simulink model "simulinkModel"  (R2021b)
settings: Solver=FixedStepAuto  StartTime=0.0  StopTime=50  FixedStep=0.05  RelTol=1e-3
model workspace (MAT data in the model file):
  R_wheel = 0.0565
  W = 0.055
  WD = 0.573125555665
  a = 0.306622172281
  b = 0.228377827719
  c = 0.38
  l = 0.535
  m = 13.4973333333
  m_LF = 2867.66666667
  m_LR = 3883.33333333
  m_RF = 2894
  m_RR = 3852.33333333
  m_f = 5761.66666667
  m_r = 7735.66666667
undefined symbols (not defined in the file or in its folder): sigbuilder_block
libraries: slpidlib x1
settings Model: PacingRate=0.100000  Creator=Mikeh  LastModifiedBy=20212181
settings DebuggingCC: SignalInfNanChecking=error

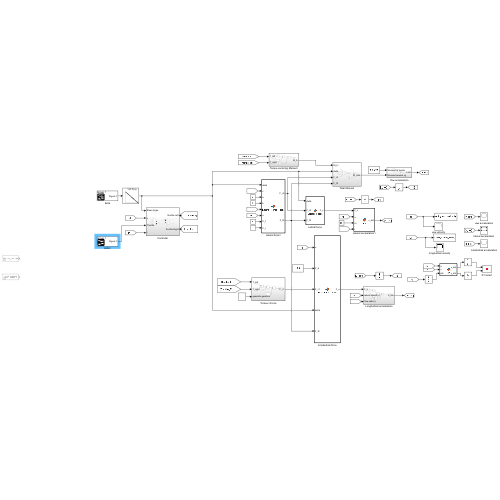
[thumbnail: Simulink's stored preview of the top-level diagram]
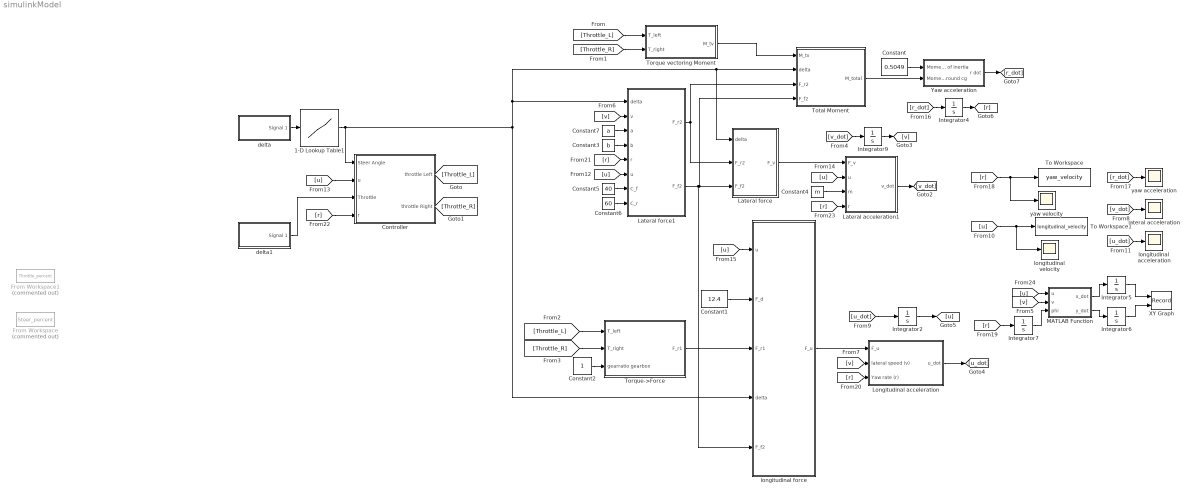
== system simulinkModel ==
  1-D Lookup Table1 : Lookup_n-D  NumberOfTableDimensions=1  BreakpointsForDimension1=[-50:50]  Table=-(([-50:50])/100)*0.4363*2  InternalRulePriority=Speed  RndMeth=Simplest  InputSameDT=on
  Constant : Constant  Value=0.5049
  Constant1 : Constant  Value=12.4
  Constant2 : Constant
  Constant3 : Constant  Value=b
  Constant4 : Constant  Value=m
  Constant5 : Constant  Value=40
  Constant6 : Constant  Value=60
  Constant7 : Constant  Value=a
  Controller : Subsystem
  From Workspace : FromWorkspace  Commented=on  VariableName=Steer_percent  OutDataTypeStr=double
  From Workspace1 : FromWorkspace  Commented=on  VariableName=Throttle_percent  OutDataTypeStr=double
  Integrator{2,4..7,9} (6 alike) : Integrator
  Lateral acceleration1 : MATLAB Function  TreatAsAtomicUnit=on
  Lateral force : MATLAB Function  TreatAsAtomicUnit=on
  Lateral force1 : MATLAB Function  TreatAsAtomicUnit=on
  Longitudinal acceleration : Subsystem
  MATLAB Function : MATLAB Function  TreatAsAtomicUnit=on
  To Workspace : ToWorkspace  VariableName=yaw_velocity  SaveFormat=Timeseries  SampleTime=-1
  To Workspace1 : ToWorkspace  VariableName=longitudinal_velocity  SaveFormat=Timeseries  SampleTime=-1
  Torque vectoring Moment : Subsystem
  Torque->Force : Subsystem
  Total Moment : Subsystem
  XY Graph : Record  FileSettingsInternal="{\"entries\":[{\"content\":{\"excelSettings\":{\"content\":{},\"type\":\"Streamout.ExcelSettings\"}},\"type\":\"Streamout.FileSettingStorage\",\"uuid\":\"f41fdb41-5409-4f7b-aadf-d421236eabc4\"}],\"packageUris\":[\"http://schema.mathworks.com/mf0/streamout_blocks/R2020a\"],\"version\":\"1.0\"}"  Layout=[1 1]  SignalsInternal="{\"entries\":[{\"content\":{\"signals\":[{\"content\":{\"blockPath\":[\"simulinkModel/XY Graph\"],\"channel\":[],\"dimensions\":[1],\"domain\":\"simulinkModel/XY Graph\",\"lineColor\":\"#a2142f\",\"plots\":[1],\"port\":1,\"sid\":[\"\"],\"signalID\":1353,\"signalName\":\"Integrator5\"},\"type\":\"RecordBlkView.Signal\",\"uuid\":\"9f89cf65-ec70-45de-bdd1-0fbdeb2aeadf\"},{\"content\":{\"blockPath\":[\"simulinkModel/XY Graph\"],\"channel\":[],\"dimensions\":[1],\"domain\":\"simulinkModel/XY Graph\",\"lineColor\":\"#139fff\",\"plots\":[1],\"port\":2,\"sid\":[\"\"],\"signalID\":1357,\"signalName\":\"Integrator6\"},\"type\":\"RecordBlkView.Signal\",\"uuid\":\"784288ff-bbec-4878-b9c7-1aeaaa1d51b9\"}]},\"type\":\"RecordBlkView.InputSignals\",\"uuid\":\"b8f6738f-3ffc-41ef-9719-2828cc63dacd\"}],\"packageUris\":[\"http://schema.mathworks.com/mf0/streamout_blocks/R2020a\"],\"version\":\"1.0\"}"  VisualizationBindings="{\"xyplotplugin\":{\"info\":[{\"series\":[{\"bindingParametersList\":[{\"parameter\":\"X-Axis\",\"signalID\":1353,\"signalName\":\"Integrator5\"},{\"parameter\":\"Y-Axis\",\"signalID\":1357,\"signalName\":\"Integrator6\"}],\"seriesID\":60949}],\"subplotID\":1}]}}"  CompatibilityTag=XY
  Yaw acceleration : Subsystem
  delta : Subsystem  Tag=STV Subsys  LoadFcn=sigbuilder_block('load');  StartFcn=sigbuilder_block('start');  StopFcn=sigbuilder_block('stop');  ClipboardFcn=sigbuilder_block('clipboard');  mask(Sigbuilder block){tuvar=[0:10]}
      mask help: Simulink:masks:SigbuilderBlock_MD
      mask init:
      | if ~strcmp(get_param(bdroot(gcbh),'SimulationStatus'),'stopped') tuvar = sigbuilder_block('maskInit'); end
      settings: CopyFcn=sigbuilder_block('copy');  DeleteFcn=sigbuilder_block('delete');  ModelCloseFcn=sigbuilder_block('modelClose');  PreSaveFcn=sigbuilder_block('preSave');  PauseFcn=sigbuilder_block('pause');  ContinueFcn=sigbuilder_block('continue');  NameChangeFcn=sigbuilder_block('namechange');  OpenFcn=sigbuilder_block('open',[511.2 133.2 550.8 400.2 ]);  CloseFcn=sigbuilder_block('close');
      mask Display: plot(0, 0, 100, 100,[2, 2, 32, 32, 2], [68, 8, 8, 68, 68],[32, 2], [38, 38], [32, 19, 2],[53, 60, 44], [32, 17, 17, 2],[16, 16, 31, 31]);txt = getActiveGroup(gcbh);text(2, 100, txt,'verticalAlignment', 'top');
  delta1 : Subsystem  Tag=STV Subsys  LoadFcn=sigbuilder_block('load',[511.2 133.2 550.8 400.2 ]);  StartFcn=sigbuilder_block('start');  StopFcn=sigbuilder_block('stop');  ClipboardFcn=sigbuilder_block('clipboard');  mask(Sigbuilder block){tuvar=[0:10]}
      mask help: Simulink:masks:SigbuilderBlock_MD
      mask init:
      | if ~strcmp(get_param(bdroot(gcbh),'SimulationStatus'),'stopped') tuvar = sigbuilder_block('maskInit'); end
      settings: CopyFcn=sigbuilder_block('copy');  DeleteFcn=sigbuilder_block('delete');  ModelCloseFcn=sigbuilder_block('modelClose');  PreSaveFcn=sigbuilder_block('preSave');  PauseFcn=sigbuilder_block('pause');  ContinueFcn=sigbuilder_block('continue');  NameChangeFcn=sigbuilder_block('namechange');  OpenFcn=sigbuilder_block('open',[511.2 133.2 550.8 400.2 ]);  CloseFcn=sigbuilder_block('close');
      mask Display: plot(0, 0, 100, 100,[2, 2, 32, 32, 2], [68, 8, 8, 68, 68],[32, 2], [38, 38], [32, 19, 2],[53, 60, 44], [32, 17, 17, 2],[16, 16, 31, 31]);txt = getActiveGroup(gcbh);text(2, 100, txt,'verticalAlignment', 'top');
  lateral acceleration : Scope
  longitudinal acceleration : Scope
  longitudinal force : MATLAB Function  TreatAsAtomicUnit=on
  longitudinal velocity : Scope
  yaw acceleration : Scope
  yaw velocity : Scope
  wires:
  Total Moment/1(M_total) -> Yaw acceleration/2(Moment around cg)
  Torque vectoring Moment/1(M_tv) -> Total Moment/1(M_tv)
  Constant4/1 -> Lateral acceleration1/3(m)
  Lateral force/1(F_v) -> Lateral acceleration1/1(F_v)
  Lateral acceleration1/1(v_dot) -> [v_dot]
  Torque->Force/1(F_r1) -> longitudinal force/3(F_r1)
  longitudinal force/1(F_u) -> Longitudinal acceleration/1(F_u)
  1-D Lookup Table1/1 -> Lateral force1/1(delta), Lateral force/1(delta), Total Moment/2(delta), longitudinal force/4(delta), Controller/1(Steer Angle)
  delta1/1(Signal 1) -> Controller/3(Throttle)
  Constant/1 -> Yaw acceleration/1(Moment of Inertia)
  Constant1/1 -> longitudinal force/2(F_d)
  Constant2/1 -> Torque->Force/3(gearratio gearbox)
  [u] -> longitudinal velocity/1, To Workspace1/1
  delta/1(Signal 1) -> 1-D Lookup Table1/1
  Lateral force1/1(F_r2) -> Lateral force/2(F_r2), Total Moment/3(F_r2)
  Lateral force1/2(F_f2) -> longitudinal force/5(F_f2), Lateral force/3(F_f2), Total Moment/4(F_f2)
  Constant3/1 -> Lateral force1/4(b)
  Constant5/1 -> Lateral force1/7(C_f)
  Constant6/1 -> Lateral force1/8(C_r)
  Constant7/1 -> Lateral force1/3(a)
  Integrator5/1 -> XY Graph/1
  MATLAB Function/2(y_dot) -> Integrator6/1
  Integrator6/1 -> XY Graph/2
  MATLAB Function/1(x_dot) -> Integrator5/1
  Integrator7/1 -> MATLAB Function/3(phi)
  [r] -> yaw velocity/1, To Workspace/1
  Controller/1(throttle Left) -> [Throttle_L]
  Controller/2(throttle Right) -> [Throttle_R]
  [Throttle_L] -> Torque vectoring Moment/1(T_left)
  [Throttle_R] -> Torque vectoring Moment/2(T_right)
  [Throttle_L] -> Torque->Force/1(T_left)
  [Throttle_R] -> Torque->Force/2(T_right)
  [v_dot] -> Integrator9/1
  Integrator9/1 -> [v]
  [v] -> MATLAB Function/2(v)
  [v] -> Lateral force1/2(v)
  [v] -> Longitudinal acceleration/2(lateral speed (v))
  [v_dot] -> lateral acceleration/1
  Longitudinal acceleration/1(u_dot) -> [u_dot]
  Integrator2/1 -> [u]
  [u_dot] -> Integrator2/1
  [u_dot] -> longitudinal acceleration/1
  [u] -> Lateral force1/6(u)
  [u] -> Controller/2(u)
  [u] -> Lateral acceleration1/2(u)
  [u] -> longitudinal force/1(u)
  [r_dot] -> Integrator4/1
  Integrator4/1 -> [r]
  Yaw acceleration/1(r dot) -> [r_dot]
  [r_dot] -> yaw acceleration/1
  [r] -> Integrator7/1
  [r] -> Longitudinal acceleration/3(Yaw rate (r))
  [r] -> Lateral force1/5(r)
  [r] -> Controller/4(r)
  [r] -> Lateral acceleration1/4(r)
  [u] -> MATLAB Function/1(u)

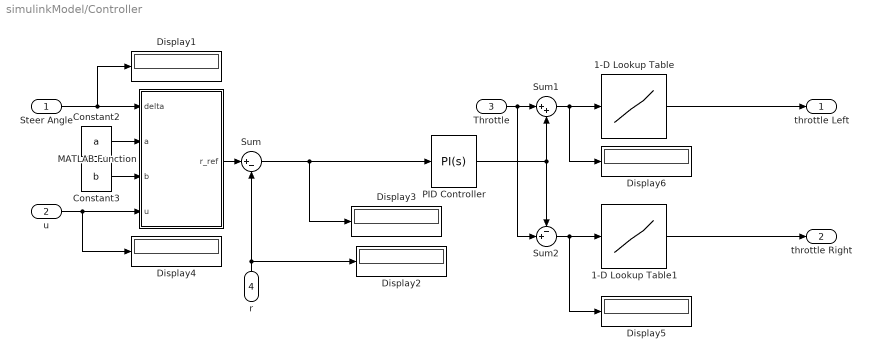
== system simulinkModel/Controller ==
  Steer Angle : Inport
  u : Inport  Port=2
  Throttle : Inport  Port=3
  r : Inport  Port=4
  1-D Lookup Table : Lookup_n-D  NumberOfTableDimensions=1  BreakpointsForDimension1=[0:100]  Table=(([0:100]-50)/100)*5.28*2  InternalRulePriority=Speed  RndMeth=Simplest  InputSameDT=on
  1-D Lookup Table1 : Lookup_n-D  NumberOfTableDimensions=1  BreakpointsForDimension1=[0:100]  Table=(([0:100]-50)/100)*5.28*2  InternalRulePriority=Speed  RndMeth=Simplest  InputSameDT=on
  Constant2 : Constant  Value=a
  Constant3 : Constant  Value=b
  Display{1..6} (6 alike) : Display
  MATLAB Function : MATLAB Function  TreatAsAtomicUnit=on
  PID Controller : slpidlib/PID Controller  Controller=PI  Form=Parallel  TimeDomain=Continuous-time  UseExternalTs=off  SampleTime=-1  IntegratorMethod=Forward Euler  FilterMethod=Forward Euler  ControllerParametersSource=internal  P=0  I=0  D=0  UseFilter=on  N=100  TunerSelectOption=Transfer Function Based (PID Tuner App)  InitialConditionSource=internal  InitialConditionForIntegrator=0  InitialConditionForFilter=0  DifferentiatorICPrevScaledInput=0  ExternalReset=none  TrackingMode=off  Kt=1  LimitOutput=off  SatLimitsSource=internal  UpperSaturationLimit=inf  LowerSaturationLimit=-inf  LinearizeAsGain=on  AntiWindupMode=none  Kb=1  POutMin=[]  POutMax=[]  IOutMin=[]  IOutMax=[]  DOutMin=[]  DOutMax=[]  NOutMin=[]  NOutMax=[]  SumOutMin=[]  SumOutMax=[]  SaturationOutMin=[]  SaturationOutMax=[]  PParamMin=[]  PParamMax=[]  IParamMin=[]  IParamMax=[]  DParamMin=[]  DParamMax=[]  NParamMin=[]  NParamMax=[]  KbParamMin=[]  KbParamMax=[]  KtParamMin=[]  KtParamMax=[]  KbOutMin=[]  KbOutMax=[]  KtOutMin=[]  KtOutMax=[]  IntegratorOutMin=[]  IntegratorOutMax=[]  FilterOutMin=[]  FilterOutMax=[]  SumI1OutMin=[]  SumI1OutMax=[]  SumI2OutMin=[]  SumI2OutMax=[]  SumI3OutMin=[]  SumI3OutMax=[]  SumI4OutMin=[]  SumI4OutMax=[]  SumDOutMin=[]  SumDOutMax=[]  DifferentiatorOutMin=[]  DifferentiatorOutMax=[]  FilterDiffOutCoefMin=[]  FilterDiffOutCoefMax=[]  ReciprocalOutMin=[]  ReciprocalOutMax=[]  SumDenOutMin=[]  SumDenOutMax=[]  SumNumOutMin=[]  SumNumOutMax=[]  DivideOutMin=[]  DivideOutMax=[]  UdiffTsProdOutMin=[]  UdiffTsProdOutMax=[]  NTsProdOutMin=[]  NTsProdOutMax=[]  UintegralTsProdOutMin=[]  UintegralTsProdOutMax=[]  UngainTsProdOutMin=[]  UngainTsProdOutMax=[]  FilterDenConstantOutDataTypeStr=Inherit: Inherit via back propagation  FilterDenConstantOutMin=[]  FilterDenConstantOutMax=[]  PCopyOutDataTypeStr=Inherit: Inherit via back propagation  PCopyOutMin=[]  PCopyOutMax=[]  NCopyOutDataTypeStr=Inherit: Inherit via back propagation  NCopyOutMin=[]  NCopyOutMax=[]  IntegratorContinuousStateAttributes=''  IntegratorStateMustResolveToSignalObject=off  IntegratorRTWStateStorageClass=Auto  FilterContinuousStateAttributes=''  FilterStateMustResolveToSignalObject=off  FilterRTWStateStorageClass=Auto  ParallelPVariant=InternalParameters  IdealPVariant=Disabled  IVariant=InternalParameters  DVariant=Disabled  IntegratorVariant=Continuous  SatVariant=Disabled  AWVariant=Passthrough  PCopyVariant=Disabled  TRVariant=Disabled  FdbkBlocksVariant=Forward  IdealPFdbkVariant=Disabled  SatFdbkVariant=Disabled  DerivativeFilterVariant=Disabled  NVariant=Disabled  NCopyVariant=Disabled_SignalSpec  FilterICVariant=Disabled  IntegratorICVariant=InternalICs  ExternalResetVariant=Disabled  TRSumVariant=Passthrough  SumFdbkVariant=Disabled  SumVariant=Sum_PI  TsampFilterVariant=InternalTs  TsampNgainVariant=Passthrough  TsampIntegralVariant=Passthrough  ExternalSaturationOutDataTypeStr=Inherit: Same as second input
  Sum : Sum  Inputs=|+-
  Sum1 : Sum  Inputs=|++
  Sum2 : Sum  Inputs=-+|
  throttle Left : Outport
  throttle Right : Outport  Port=2
  wires:
  Constant3/1 -> MATLAB Function/3(b)
  Constant2/1 -> MATLAB Function/2(a)
  Throttle/1 -> Sum2/2, Sum1/1
  u/1 -> Display4/1, MATLAB Function/4(u)
  PID Controller/1 -> Sum1/2, Sum2/1
  Steer Angle/1 -> Display1/1, MATLAB Function/1(delta)
  r/1 -> Display2/1, Sum/2
  MATLAB Function/1(r_ref) -> Sum/1
  Sum/1 -> Display3/1, PID Controller/1
  1-D Lookup Table/1 -> throttle Left/1
  Sum1/1 -> Display6/1, 1-D Lookup Table/1
  1-D Lookup Table1/1 -> throttle Right/1
  Sum2/1 -> Display5/1, 1-D Lookup Table1/1

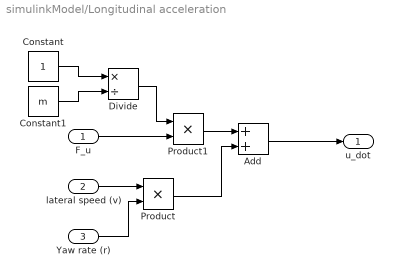
== system simulinkModel/Longitudinal acceleration ==
  F_u : Inport
  lateral speed (v) : Inport  Port=2
  Yaw rate (r) : Inport  Port=3
  Add : Sum
  Constant : Constant
  Constant1 : Constant  Value=m
  Divide : Product  Inputs=*/
  Product : Product
  Product1 : Product
  u_dot : Outport
  wires:
  Constant/1 -> Divide/1
  Constant1/1 -> Divide/2
  lateral speed (v)/1 -> Product/1
  Yaw rate (r)/1 -> Product/2
  F_u/1 -> Product1/2
  Divide/1 -> Product1/1
  Product1/1 -> Add/1
  Product/1 -> Add/2
  Add/1 -> u_dot/1

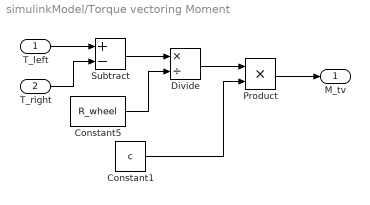
== system simulinkModel/Torque vectoring Moment ==
  T_left : Inport
  T_right : Inport  Port=2
  Constant1 : Constant  Value=c
  Constant5 : Constant  Value=R_wheel
  Divide : Product  Inputs=*/
  Product : Product
  Subtract : Sum  Inputs=+-
  M_tv : Outport
  wires:
  T_left/1 -> Subtract/1
  T_right/1 -> Subtract/2
  Subtract/1 -> Divide/1
  Constant5/1 -> Divide/2
  Divide/1 -> Product/1
  Constant1/1 -> Product/2
  Product/1 -> M_tv/1

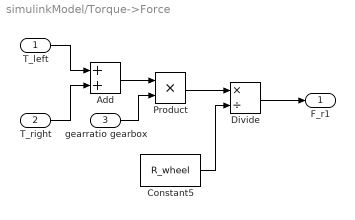
== system simulinkModel/Torque->Force ==
  T_left : Inport
  T_right : Inport  Port=2
  gearratio gearbox : Inport  Port=3
  Add : Sum
  Constant5 : Constant  Value=R_wheel
  Divide : Product  Inputs=*/
  Product : Product
  F_r1 : Outport
  wires:
  T_left/1 -> Add/1
  T_right/1 -> Add/2
  Add/1 -> Product/1
  gearratio gearbox/1 -> Product/2
  Product/1 -> Divide/1
  Constant5/1 -> Divide/2
  Divide/1 -> F_r1/1

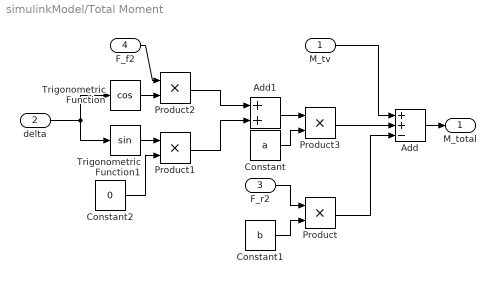
== system simulinkModel/Total Moment ==
  M_tv : Inport
  delta : Inport  Port=2
  F_r2 : Inport  Port=3
  F_f2 : Inport  Port=4
  Add : Sum  Inputs=++-
  Add1 : Sum
  Constant : Constant  Value=a
  Constant1 : Constant  Value=b
  Constant2 : Constant  Value=0
  Product{,1..3} (4 alike) : Product
  Trigonometric Function : Trigonometry  Operator=cos
  Trigonometric Function1 : Trigonometry
  M_total : Outport
  wires:
  Constant1/1 -> Product/2
  F_r2/1 -> Product/1
  Add/1 -> M_total/1
  Product/1 -> Add/3
  M_tv/1 -> Add/1
  delta/1 -> Trigonometric Function1/1, Trigonometric Function/1
  Trigonometric Function1/1 -> Product1/1
  Constant2/1 -> Product1/2
  Trigonometric Function/1 -> Product2/2
  F_f2/1 -> Product2/1
  Product2/1 -> Add1/1
  Product1/1 -> Add1/2
  Add1/1 -> Product3/1
  Product3/1 -> Add/2
  Constant/1 -> Product3/2

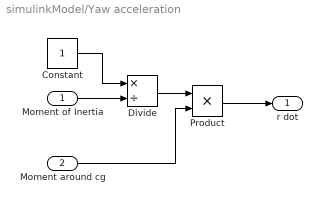
== system simulinkModel/Yaw acceleration ==
  Moment of Inertia : Inport
  Moment around cg : Inport  Port=2
  Constant : Constant
  Divide : Product  Inputs=*/
  Product : Product
  r dot : Outport
  wires:
  Moment of Inertia/1 -> Divide/2
  Constant/1 -> Divide/1
  Divide/1 -> Product/1
  Moment around cg/1 -> Product/2
  Product/1 -> r dot/1

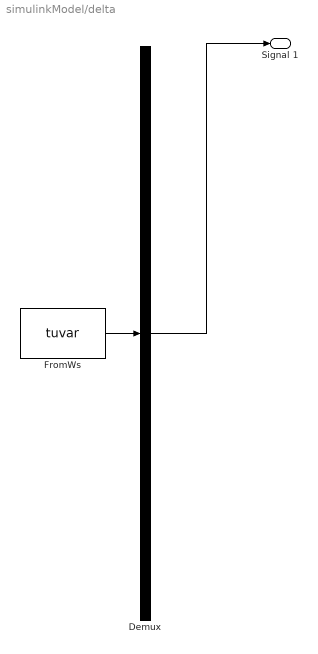
== system simulinkModel/delta ==
  Demux : Demux  Tag=STV Demux  Outputs=1
      settings: DisplayOption=none
  FromWs : FromWorkspace  Tag=STV FromWs  VariableName=tuvar
      SigBuilderData=|
      | common.afterFinalStr = 'Extrapolate'
      | common.sampleTime = 0
      | dataSet.timeRange = [0 10]
      | dataSet.name = 'Group 1'
      | sbobj.Groups.Name = 'Group 1'
      | sbobj.Groups.Signals.Name = 'Signal 1'
      | sbobj.Groups.Signals.XData = [0 10]
      | sbobj.Groups.Signals.YData = [-40 -40]
  Signal 1 : Outport  Tag=STV Outport
  wires:
  Demux/1 -> Signal 1/1
  FromWs/1 -> Demux/1

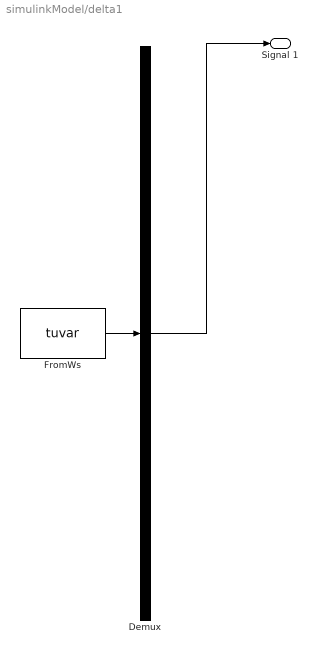
== system simulinkModel/delta1 ==
  Demux : Demux  Tag=STV Demux  Outputs=1
      settings: DisplayOption=none
  FromWs : FromWorkspace  Tag=STV FromWs  VariableName=tuvar
      SigBuilderData=|
      | common.afterFinalStr = 'Extrapolate'
      | common.sampleTime = 0
      | dataSet.timeRange = [0 50]
      | dataSet.name = 'Group 1'
      | sbobj.Groups.Name = 'Group 1'
      | sbobj.Groups.Signals.Name = 'Signal 1'
      | sbobj.Groups.Signals.XData = [0 50]
      | sbobj.Groups.Signals.YData = [50 56]
      | sbobj.Groups.TimeRange = [0 50]
  Signal 1 : Outport  Tag=STV Outport
  wires:
  Demux/1 -> Signal 1/1
  FromWs/1 -> Demux/1

== matlab function simulinkModel/Lateral acceleration1 ==
  data: F_v input; u input; v_dot output; m input; r input
function v_dot = fcn(F_v, u, m, r)
v_dot = double((1/m)*F_v - u *r);

== matlab function simulinkModel/Lateral force ==
  data: delta input; F_v output; F_r2 input; F_f2 input
function F_v = Lateral_Force(delta, F_r2, F_f2)
F_v = F_r2 + cos(delta)*F_f2;

== matlab function simulinkModel/longitudinal force ==
  data: u input; F_d input; F_r1 input; delta input; F_f2 input; F_u output
function F_u = longitudinal_force(u,F_d,F_r1, delta, F_f2)
if u>0
    F_dreal = F_d;
elseif u<0
    F_dreal = -F_d;
else
    F_dreal = 0;
end
F_u = F_r1 - sin(delta)*F_f2 - F_dreal;

== matlab function simulinkModel/Controller/MATLAB Function ==
  data: delta input; a input; b input; u input; r_ref output
function r_ref = r(delta,a,b,u)
r_ref = ((tan(delta))/(a+b)) * u;

== matlab function simulinkModel/Lateral force1 ==
  data: F_r2 output; delta input; F_f2 output; v input; a input; b input; r input; u input; C_f input; C_r input
function [F_r2,F_f2] = Lateral_Force_Front(delta,v,a,b,r,u, C_f,C_r)
if abs(u)>0
    alpha_r = atan((-v+b*r)/u);
    alpha_f = delta + atan((-v-a*r)/u);
else
    alpha_r = 0;
    alpha_f = 0;
end

F_f2 = C_f*alpha_f;
F_r2 = C_r*alpha_r;

== matlab function simulinkModel/MATLAB Function ==
  data: u input; x_dot output; v input; phi input; y_dot output
function [x_dot, y_dot] = fcn(u, v, phi)

x_dot = u*cos(phi) - v*sin(phi);
y_dot = u*sin(phi) + v*cos(phi);
